simulink library "jailib"  (R2013a)
settings: Solver=ode45  StartTime=0.0  StopTime=10.0  RelTol=1e-3
libraries: powerlib x11
settings Model: Creator=ChakZ  LastModifiedBy=ChakZ

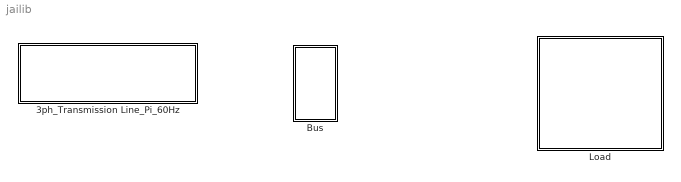
== system jailib ==
  3ph_Transmission Line_Pi_60Hz : Subsystem  mask{R=0.0085, X=0, B=0, MVA=100, KV=230}
      mask prompts: R "Resistance (pu)"; X "Reactance(pu)"; B "Susceptance (pu)(B/2)"; MVA "MVA Base"; KV "KV Base"
      mask help: Transmission Line Pi model
      mask init:
      | rt = R*(KV^2)/MVA;
      | lt = (X/377)*(KV^2)/MVA;
      | ct = (2*B/377)/((KV^2)/MVA);
      | ro = 2.5*R*(KV^2)/MVA;
      | lo = 2.5*(X/377)*(KV^2)/MVA;
      | co = (2*B/377)/((1.6*KV^2)/MVA);
      mask Display:
      | patch([0.0 0.0 1 1 0.0 0.0 ],[0.4 0.7 0.7 0.4 0.4 0.7],[0 0 1]);
      | patch([0.4 0.4 0.42 0.42],[0.4 0.75 0.75 0.4],[1 0 0]);
      | patch([0.38 0.38 0.57 0.57],[0.7 0.75 0.75 0.7],[1 0 0]);
      | patch([0.53 0.53 0.55 0.55],[0.4 0.75 0.75 0.4],[1 0 0]);
  Bus : Subsystem
  Load : Subsystem
      mask Display:
      | patch([0 0.5 1 0],[1 0 1 1],[1 1 0]);
      | color('red');
      | plot([0.1 0.5 0.9 0.1],[0.9 0.1 0.9 0.9]);

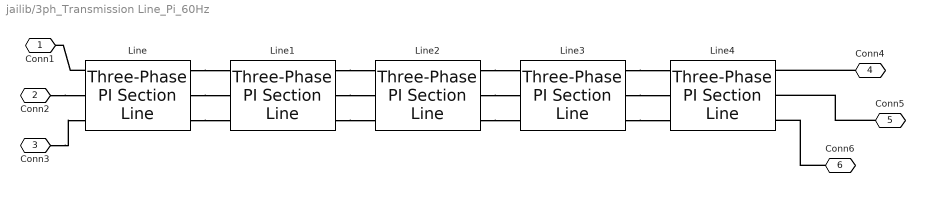
== system jailib/3ph_Transmission Line_Pi_60Hz ==
  Line{,1..4} (5 alike) : powerlib/Elements/Three-Phase PI Section Line  LConnTagsString=a|b|c  RConnTagsString=A|B|C  Frequency=60  Resistances=[rt ro] /100  Inductances=[ lt lo] /100  Capacitances=[ct co]/100  Length=20
  Conn1 : PMIOPort  Port=1  Side=Left
  Conn2 : PMIOPort  Port=2  Side=Left
  Conn3 : PMIOPort  Port=3  Side=Left
  Conn4 : PMIOPort  Port=4  Side=Right
  Conn5 : PMIOPort  Port=5  Side=Right
  Conn6 : PMIOPort  Port=6  Side=Right
  connections:
  Conn5/RConn1 -- Line4/RConn2
  Conn2/RConn1 -- Line/LConn2
  Conn4/RConn1 -- Line4/RConn1
  Conn6/RConn1 -- Line4/RConn3
  Line/LConn1 -- Conn1/RConn1
  Conn3/RConn1 -- Line/LConn3
  Line/RConn1 -- Line1/LConn1
  Line1/RConn2 -- Line2/LConn2
  Line3/RConn2 -- Line4/LConn2
  Line3/RConn1 -- Line4/LConn1
  Line1/RConn1 -- Line2/LConn1
  Line2/RConn2 -- Line3/LConn2
  Line/RConn2 -- Line1/LConn2
  Line1/RConn3 -- Line2/LConn3
  Line2/RConn1 -- Line3/LConn1
  Line2/RConn3 -- Line3/LConn3
  Line/RConn3 -- Line1/LConn3
  Line3/RConn3 -- Line4/LConn3

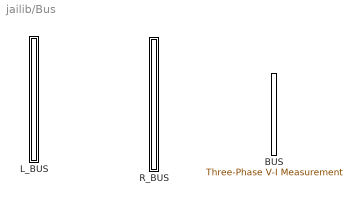
== system jailib/Bus ==
  BUS : powerlib/Measurements/Three-Phase V-I Measurement  VoltageMeasurement=phase-to-ground  SetLabelV=on  LabelV=Vabc  Vpu=on  VpuLL=off  CurrentMeasurement=yes  SetLabelI=on  LabelI=Iabc  Ipu=on  Pbase=100e6  Vbase=13.8e3  OutputType=Complex  PhasorSimulation=off  PSBequivalent=0
  L_BUS : Subsystem  mask{K=on}
      mask prompts: K "KV"
  R_BUS : Subsystem  mask{K=on}
      mask prompts: K "KV"

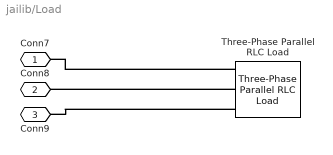
== system jailib/Load ==
  Three-Phase Parallel RLC Load : powerlib/Elements/Three-Phase Parallel RLC Load  LConnTagsString=A|B|C  Configuration=Y (grounded)  NominalVoltage=(230000)*1.01315  NominalFrequency=60  ActivePower=90e6  InductivePower=30e6  CapacitivePower=0  Measurements=None  LoadType=constant PQ
  Conn7 : PMIOPort  Port=1  Side=Left
  Conn8 : PMIOPort  Port=2  Side=Left
  Conn9 : PMIOPort  Port=3  Side=Left
  connections:
  Three-Phase Parallel RLC Load/LConn1 -- Conn7/RConn1
  Three-Phase Parallel RLC Load/LConn2 -- Conn8/RConn1
  Three-Phase Parallel RLC Load/LConn3 -- Conn9/RConn1

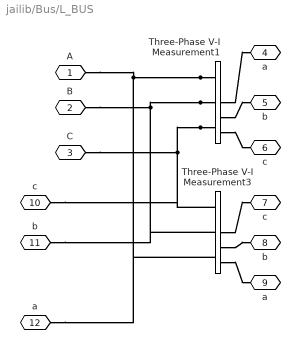
== system jailib/Bus/L_BUS ==
  Three-Phase V-I Measurement1 : powerlib/Measurements/Three-Phase V-I Measurement  VoltageMeasurement=phase-to-ground  SetLabelV=on  LabelV=Vabc_7  Vpu=on  VpuLL=off  CurrentMeasurement=yes  SetLabelI=on  LabelI=Iabc_7  Ipu=on  Pbase=100e6  Vbase=230e3  OutputType=Complex  PhasorSimulation=off  PSBequivalent=0
  Three-Phase V-I Measurement3 : powerlib/Measurements/Three-Phase V-I Measurement  VoltageMeasurement=phase-to-ground  SetLabelV=on  LabelV=Vab  Vpu=on  VpuLL=off  CurrentMeasurement=yes  SetLabelI=on  LabelI=Iab  Ipu=on  Pbase=100e6  Vbase=230e3  OutputType=Complex  PhasorSimulation=off  PSBequivalent=0
  A : PMIOPort  Port=1  Side=Left
  B : PMIOPort  Port=2  Side=Left
  C : PMIOPort  Port=3  Side=Left
  a : PMIOPort  Port=4  Side=Right
  b : PMIOPort  Port=5  Side=Right
  c : PMIOPort  Port=6  Side=Right
  "c " : PMIOPort  Port=7  Side=Right
  "b " : PMIOPort  Port=8  Side=Right
  "a " : PMIOPort  Port=9  Side=Right
  "c  " : PMIOPort  Port=10  Side=Left
  "b  " : PMIOPort  Port=11  Side=Left
  "a  " : PMIOPort  Port=12  Side=Left
  connections:
  Three-Phase V-I Measurement1/LConn3 -- "c  "/RConn1 -- Three-Phase V-I Measurement3/LConn1 -- C/RConn1
  Three-Phase V-I Measurement1/LConn2 -- "b  "/RConn1 -- Three-Phase V-I Measurement3/LConn2 -- B/RConn1
  Three-Phase V-I Measurement1/LConn1 -- A/RConn1 -- "a  "/RConn1 -- Three-Phase V-I Measurement3/LConn3
  Three-Phase V-I Measurement3/RConn3 -- "a "/RConn1
  Three-Phase V-I Measurement1/RConn3 -- c/RConn1
  Three-Phase V-I Measurement1/RConn1 -- a/RConn1
  Three-Phase V-I Measurement1/RConn2 -- b/RConn1
  Three-Phase V-I Measurement3/RConn1 -- "c "/RConn1
  Three-Phase V-I Measurement3/RConn2 -- "b "/RConn1

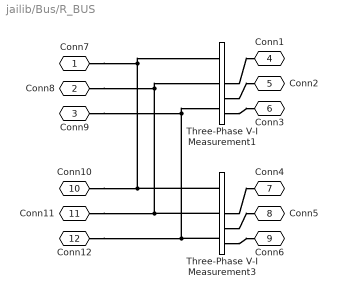
== system jailib/Bus/R_BUS ==
  Three-Phase V-I Measurement1 : powerlib/Measurements/Three-Phase V-I Measurement  VoltageMeasurement=phase-to-ground  SetLabelV=on  LabelV=Vabc_9  Vpu=on  VpuLL=off  CurrentMeasurement=yes  SetLabelI=on  LabelI=Iabc_9  Ipu=on  Pbase=100e6  Vbase=230e3  OutputType=Complex  PhasorSimulation=off  PSBequivalent=0
  Three-Phase V-I Measurement3 : powerlib/Measurements/Three-Phase V-I Measurement  VoltageMeasurement=phase-to-ground  SetLabelV=on  LabelV=Vabc  Vpu=on  VpuLL=off  CurrentMeasurement=yes  SetLabelI=on  LabelI=Iabc  Ipu=on  Pbase=100e6  Vbase=230e3  OutputType=Complex  PhasorSimulation=off  PSBequivalent=0
  Conn7 : PMIOPort  Port=1  Side=Left
  Conn8 : PMIOPort  Port=2  Side=Left
  Conn9 : PMIOPort  Port=3  Side=Left
  Conn1 : PMIOPort  Port=4  Side=Right
  Conn2 : PMIOPort  Port=5  Side=Right
  Conn3 : PMIOPort  Port=6  Side=Right
  Conn4 : PMIOPort  Port=7  Side=Right
  Conn5 : PMIOPort  Port=8  Side=Right
  Conn6 : PMIOPort  Port=9  Side=Right
  Conn10 : PMIOPort  Port=10  Side=Left
  Conn11 : PMIOPort  Port=11  Side=Left
  Conn12 : PMIOPort  Port=12  Side=Left
  connections:
  Conn12/RConn1 -- Three-Phase V-I Measurement3/LConn3 -- Conn9/RConn1 -- Three-Phase V-I Measurement1/LConn3
  Conn11/RConn1 -- Three-Phase V-I Measurement3/LConn2 -- Conn8/RConn1 -- Three-Phase V-I Measurement1/LConn2
  Conn10/RConn1 -- Three-Phase V-I Measurement3/LConn1 -- Conn7/RConn1 -- Three-Phase V-I Measurement1/LConn1
  Three-Phase V-I Measurement3/RConn3 -- Conn6/RConn1
  Three-Phase V-I Measurement1/RConn3 -- Conn3/RConn1
  Three-Phase V-I Measurement1/RConn1 -- Conn1/RConn1
  Three-Phase V-I Measurement1/RConn2 -- Conn2/RConn1
  Three-Phase V-I Measurement3/RConn1 -- Conn4/RConn1
  Three-Phase V-I Measurement3/RConn2 -- Conn5/RConn1
